simulink model "single_engine_neural_260120"  (R2018b)
settings: Solver=VariableStepAuto  StartTime=0.0  StopTime=10.0  RelTol=1e-3
libraries: neural x3
settings Model: Creator=Paweł Tymiński  LastModifiedBy=Paweł Tymiński

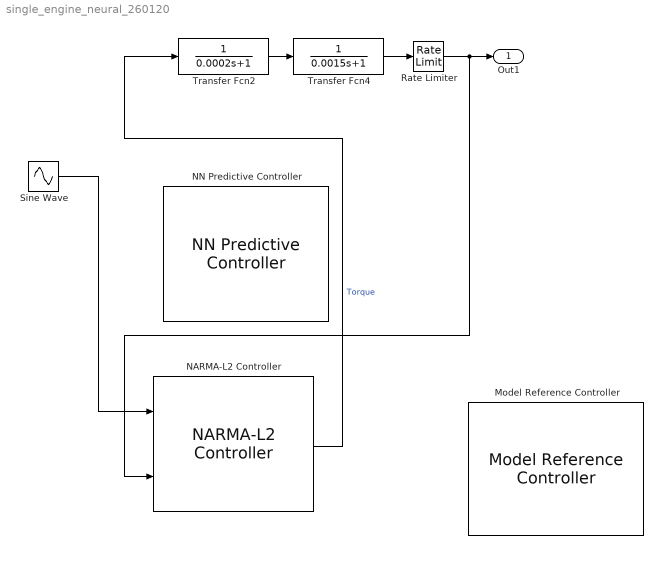
== system single_engine_neural_260120 ==
  Model Reference Controller : neural/Control Systems/Model Reference Controller  Nrc=[]  Nic=[]  Njc=[]  IW_y=[]  IW_u=[]  IW_r=[]  B1_c=[]  B2_c=[]  LW_c=[]  retraining_c=[]  max_i_int=[]  min_i_int=[]  max_r_int=[]  min_r_int=[]  Ts=[]  S1=[]  Ni=[]  Nj=[]  sim_file=0  trainfun=trainlm  Use_validation=[]  Use_Testing=[]  Use_Inc_training=[]  Use_previous_weights=[]  max_i=[]  min_i=[]  max_r=[]  min_r=[]  sam_training=[]  sam_training_c=[]  epochs=[]  epochs_c=[]  minp=[]  maxp=[]  mint=[]  maxt=[]  Normalize=[]  IW=[]  LW1_2=[]  LW2_1=[]  B1=[]  B2=[]  S1c=[]  Limit_output=[]  min_output=[]  max_output=[]  Ref_file=0
      settings: SourceProductName=Neural Network Toolbox  SourceProductBaseCode=NN
  NARMA-L2 Controller : neural/Control Systems/NARMA-L2 Controller  Normalize=0  IW1_1=[-0.84907289409835973171 1.5126044092574937316;-1.7147153340299707835 -0.21020561238515578228;1.4785922808150917529 0.91234998555658031183;1.1719784141866409488 -0.91394881896847046665;-1.2859862355485991436 -0.64207234534069901333;-0.48808133802388931066 -0.23029891949144548624;-0.37696300410323280161 1.7595650339763173609;-1.7266237346070940628 0.88876775435030863637;1.3610782383520632077 -1.1299967943100739376;-0.82244219232904980377 1.6057364275641015094]  IW3_2=[-0.49636710835342789938 -1.6258772479860281734;-0.56686104052681463017 1.8122699014348686575;-1.4967907333077721255 1.0317564827514409398;-1.6773666753889513448 0.80973784827443062717;-1.4347055255186329514 1.2363080597565876406;-0.73783979264872112669 -1.629764357371745076;1.0927320895264598377 1.2642432779317556157;1.7886845683176910704 -0.30281396818423117479;1.5822102415466958725 -0.87097424130753431371;-0.16595129548017256704 -1.7498469718752980295]  IW5_3=-0.71107373714373711682  LW2_1=[-0.25581258557879027471 -0.54152959366484632042 0.26218009482723397818 1.0921209083228975434 -0.19115378329706322891 -1.1540921214851138643 -0.16409227213024876746 -0.48815405387741056531 -0.097490136730817605892 -0.067533944558128902735]  LW4_3=[-0.41181826429018186797 -0.6479075458809432364 -0.061841422346839182433 0.57433228007474057542 1.1724372751539646753 0.044620240948435530015 0.45017153195365977592 0.34415107891727958478 1.4690602641716126175 0.076949317688849050434]  LW5_4=0.26902072699801221622  LW6_5=-0.48881553062787974628  LW6_2=0.780343302232775482  B1=[4.4667517916692922597;3.4429946958577533067;-2.3524593291502333692;-0.79427102984779851536;0.71067527043163769562;-0.71678333192309995336;-1.6145113922452387634;-1.9373675475733855844;3.4645140769249413992;-4.4329606664442602337]  B2=0.58744781590553030171  B3=[4.4197928786959943537;3.4189877086792193062;2.4268873899102678671;1.2066597091343291837;0.42028763966937093821;-0.45213055977827870668;1.535004160505305304;2.1869085463704660555;3.4333631530202826099;-4.3817533044177041646]  B4=0.93219687195387956891  Limit_output=0  min_output=0  max_output=0  Use_Previous_Weights=1  Ts=0.01  S1=10  Ni=1  Nj=2  sim_file=0  trainfun=trainlm  Use_validation=1  Use_Testing=1  max_i=3  min_i=-3  max_i_int=0  min_i_int=0  sam_training=0  epochs=25  minp=-2.455060285275362908  maxp=2.495947464788551784  mint=-2.4550602852753495853  maxt=2.495947464788551784
      settings: SourceProductName=Neural Network Toolbox  SourceProductBaseCode=NN
  NN Predictive Controller : neural/Control Systems/NN Predictive Controller  epochs=25  minp=-2.455060285275362908  maxp=2.495947464788551784  mint=-2.4550602852753495853  maxt=2.495947464788551784  Normalize=0  IW=[0.15374396783939078825 0.50808758518597185727;-0.013077929304424916121 -0.1101592463517281073;0.050603730065381484493 -0.28339520209345037127;-0.0017142951111837631626 -0.11859979777405738055;0.52388027160626471357 0.63711953454547898268;-0.0050059016001582860161 -0.11881150863444056576;-0.015756548933110101768 -0.23384167901687361035;-0.012481573847082752179 -0.10124539684703089126;0.31704169885722005562 -0.74449517497973149993;0.0055304140134286826347 -0.21550788626010558557]  LW1_2=[0.38049093261384825393 0.43152657604745442432 0.17044211539705347858 -0.10025987463497340602 -0.047756401865715315813;-0.2360311215613163649 0.057362346038914206747 -0.038612665371176163598 0.049408936862354667363 -0.010654587897251092954;-0.35507035608074399846 0.0085239157351332753981 0.029739957282679384265 -0.00032632817835834704995 -0.0090084455889577388227;-0.26030337138345671644 0.06126469657857532003 0.0052146224080525348243 0.0060400903525787636231 0.0083564726536189733869;0.47954308283808594338 0.17973910227453582245 0.13133613804098698274 0.15612529367737329467 -0.51085082002758919195;-0.09338882163175594997 -0.0088175685810721604607 -0.052632443055452400593 0.026050454948111131936 -0.028121670243573423237;-0.47246859036533700449 0.18741520162972191699 0.11436913488955816054 -0.47888988559665601752 -0.10241007512680164182;-0.30022922583673233854 0.074791759676501493037 0.24331141968603459125 -0.37840970594632711288 0.16769162704662851637;-0.76929970212597265089 0.42430894015193160174 0.045737834598177762313 0.26795077106710618597 0.4082109607427508724;-0.26670220212131723336 0.018324750131121645552 -0.019529570481191197567 0.0021756402590066147192 -0.0061176054499289126212]  LW2_1=[-0.019452205446297970992 -1.2575100781998052035 -0.32107664434298788247 -1.6905676823169559775 0.00063911921655958824594 -0.81270536878793731006 -0.016644657879900180697 -0.21514301469964755564 0.0067598565850933624993 -0.95303551413796561143]  B1=[-2.0544145324145008935;0.8343531744730400268;1.3106174250392172986;-0.41739286854875562449;-0.32467416399666848559;0.23395450678603058048;-0.78138887566137271712;0.69989781171922660352;-1.5387162115131987061;-1.7020468562805786128]  B2=-0.12936641119864897287  max_i_int=0  min_i_int=0  limit_output=0  max_output=0  min_output=0  Use_Previous_Weights=1  N2=7  Nu=2  Ts=0.01  rho=0.5  alpha=1  csrchfun=csrchbac  maxiter=1  S1=10  Ni=2  Nj=5  sim_file=0  trainfun=trainlm  Use_validation=1  Use_Testing=1  max_i=3  min_i=-3  sam_training=0
      settings: SourceProductName=Neural Network Toolbox  SourceProductBaseCode=NN
  Rate Limiter : RateLimiter  RisingSlewLimit=18.5  FallingSlewLimit=-18.5  SampleTimeMode=inherited
  Sine Wave : Sin  SampleTime=0
  Transfer Fcn2 : TransferFcn  Denominator=[0.0002 1]
  Transfer Fcn4 : TransferFcn  Denominator=[0.0015 1]
  Out1 : Outport
  wires:
  Rate Limiter/1 -> NARMA-L2 Controller/2, Out1/1
  Transfer Fcn4/1 -> Rate Limiter/1
  Transfer Fcn2/1 -> Transfer Fcn4/1
  Sine Wave/1 -> NARMA-L2 Controller/1
  NARMA-L2 Controller/1 -> Transfer Fcn2/1  "Torque"
